simulink model "model_sample17a"  (R2017a)
settings: Solver=ode4  StartTime=0.0  StopTime=1000  FixedStep=1/30  RelTol=1e-3  EnableMultiTasking=on
settings Model: SimulationMode=external  ExtModeTrigDuration=200000  Creator=krecmich  LastModifiedBy=gurtnmar
settings DataIOCC: LimitDataPoints=on  SaveFormat=Array
settings OptimizationCC: ExpressionDepthLimit=2147483647  LifeSpan=1
settings DebuggingCC: UnderspecifiedInitializationDetection=Classic  MergeDetectMultiDrivingBlocksExec=none  SolverPrmCheckMsg=warning  StateNameClashWarn=warning  SFUnexpectedBacktrackingDiag=warning  SFNoUnconditionalDefaultTransitionDiag=warning  SFExecutionAtInitializationDiag=none
settings HardwareCC: ProdBitPerLong=64  ProdLargestAtomicFloat=None  ProdHWDeviceType=Intel->x86-64
settings ModelReferenceCC: PropagateSignalLabelsOutOfModel=off
settings SFSimCC: MATLABDynamicMemAlloc=off
settings RTWCC: SystemTargetFile=ert_linux.tlc  MakeCommand="make_rtw OPT_OPTS=\"-O2 -ggdb -Wall\" CC=aarch64-linux-gnu-gcc CPP=aarch64-linux-gnu-gcc"  TemplateMakefile=ert_linux.tmf  Description=Linux Embedded Coder
settings CodeAppCC: IgnoreCustomStorageClasses=off  CustomSymbolStrType=$N$R$M  InternalIdentifier=Classic
settings STFCustomTargetCC: TargetLangStandard=C99 (ISO)  ModelReferenceCompliant=off  CombineOutputUpdateFcns=on  ERTCustomFileBanners=on  RemoveResetFunc=on  MATLABClassNameForMDSCustomization=Simulink.SoftwareTarget.ERTCustomization  GRTInterface=off  SystemTargetFile=ert_linux.tlc
settings ERTTargetCC: TargetLangStandard=C99 (ISO)  MultiwordLength=2048  ModelReferenceCompliant=off  ParMdlRefBuildCompliant=off  CompOptLevelCompliant=off  ConcurrentExecutionCompliant=off  ERTFirstTimeCompliant=off  SupportContinuousTime=on  SupportNonInlinedSFcns=on  ModelStepFunctionPrototypeControlCompliant=off  CPPClassGenCompliant=off  UseToolchainInfoCompliant=off  ExtMode=on  ExtModeMexArgs='147.32.86.138'  ERTCustomFileTemplate=ert_linux_file_process.tlc  ConvertIfToSwitch=off  SuppressUnreachableDefaultCases=off
settings ConfigComp: CovMetricSettings=dw  CovHtmlReporting=on  CovSaveCumulativeToWorkspaceVar=on  CovSaveSingleToWorkspaceVar=on  CovExternalEMLEnable=off

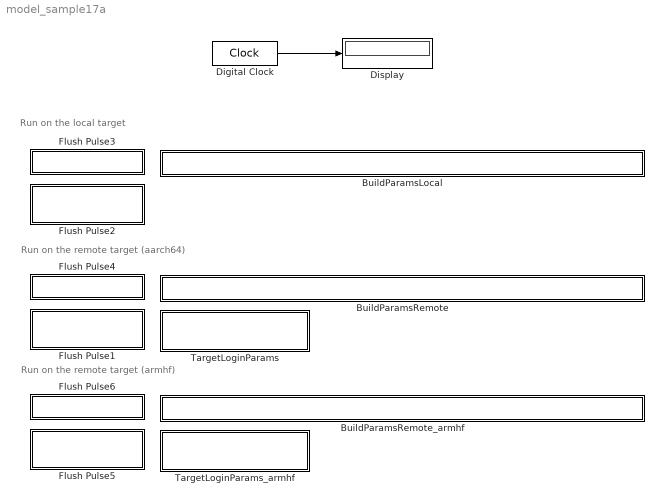
== system model_sample17a ==
  note: Run on the local target
  note: Run on the remote target (aarch64)
  note: Run on the remote target (armhf)
  BuildParamsLocal : Subsystem  mask{make_command='make_rtw OPT_OPTS="-O2 -ggdb -Wall" CC=gcc'}
      mask prompts: make_command "MakeCommand"
      mask Display: disp(get_param(gcb, 'make_command'));
  BuildParamsRemote : Subsystem  mask{make_command='make_rtw OPT_OPTS="-O2 -ggdb -Wall" CC=aarch64-linux-gnu-gcc CPP=aarch64-linux-gnu-gcc'}
      mask prompts: make_command "MakeCommand"
      mask Display: disp(get_param(gcb, 'make_command'));
  BuildParamsRemote_armhf : Subsystem  mask{make_command='make_rtw OPT_OPTS="-O2 -ggdb -Wall" CC=arm-linux-gnueabihf-gcc CPP=arm-linux-gnueabihf-gcc'}
      mask prompts: make_command "MakeCommand"
      mask Display: disp(get_param(gcb, 'make_command'));
  Digital Clock : DigitalClock
  Display : Display
  Flush Pulse1 : Subsystem
      settings: OpenFcn=|
      | % get the login credentials from the TargetLoginParams block
      | trgt_ip = get_param(strcat(gcs, '/TargetLoginParams'), 'trgt_ip_addr');
      | trgt_user = get_param(strcat(gcs, '/TargetLoginParams'), 'trgt_username');
      | 
      | % Set the IP address of the target
      | set_param(getActiveConfigSet(gcs), 'ExtModeMexArgs', trgt_ip);
      | 
      | system(['./run_model.sh ', get_param(bdroot(gcbh),'name'),' ',trgt_ip,' ',trgt_user]);
      mask Display: disp('Deploy and\nwait for connection')
  Flush Pulse2 : Subsystem
      settings: OpenFcn=|
      | configSet = getActiveConfigSet(gcs);
      | % Set the make command params
      | set_param( configSet, 'MakeCommand', '''make_rtw OPT_OPTS="-O2 -ggdb -Wall" CC=gcc''')
      | 
      | % Set the IP address of the target to the localhost
      | set_param(getActiveConfigSet(gcs), 'ExtModeMexArgs', '''127.0.0.1''')
      | 
      | system(['./run_model.sh ', get_param(bdroot(gcbh),'name')]);
      mask Display: disp('Deploy and\nwait for connection')
  Flush Pulse3 : Subsystem
      settings: OpenFcn=|
      | configSet = getActiveConfigSet(gcs);
      | % Set the make command params
      | set_param( configSet, 'MakeCommand', eval(get_param(strcat(gcs, '/BuildParamsLocal'), 'make_command')))
      | 
      | % Build the model
      | rtwbuild(gcs);
      mask Display: disp('Build')
  Flush Pulse4 : Subsystem
      settings: OpenFcn=|
      | configSet = getActiveConfigSet(gcs);
      | % Set the make command params
      | set_param( configSet, 'MakeCommand', eval(get_param(strcat(gcs, '/BuildParamsRemote'), 'make_command')))
      | 
      | % Build the model
      | rtwbuild(gcs);
      mask Display: disp('Build')
  Flush Pulse5 : Subsystem
      settings: OpenFcn=|
      | % get the login credentials from the TargetLoginParams block
      | trgt_ip = get_param(strcat(gcs, '/TargetLoginParams_armhf'), 'trgt_ip_addr');
      | trgt_user = get_param(strcat(gcs, '/TargetLoginParams_armhf'), 'trgt_username');
      | 
      | % Set the IP address of the target
      | set_param(getActiveConfigSet(gcs), 'ExtModeMexArgs', trgt_ip);
      | 
      | system(['./run_model.sh ', get_param(bdroot(gcbh),'name'),' ',trgt_ip,' ',trgt_user]);
      mask Display: disp('Deploy and\nwait for connection')
  Flush Pulse6 : Subsystem
      settings: OpenFcn=|
      | configSet = getActiveConfigSet(gcs);
      | % Set the make command params
      | set_param( configSet, 'MakeCommand', eval(get_param(strcat(gcs, '/BuildParamsRemote_armhf'), 'make_command')))
      | 
      | % Build the model
      | rtwbuild(gcs);
      mask Display: disp('Build')
  TargetLoginParams : Subsystem  mask{trgt_ip_addr='192.168.1.10', trgt_username='user'}
      mask prompts: trgt_ip_addr "Target IP address"; trgt_username "Target username"
      mask Display:
      | ip_addr = get_param(gcb, 'trgt_ip_addr');
      | user = get_param(gcb, 'trgt_username');
      | 
      | fprintf('IP addr:\t %s\n User:\t %s ', ip_addr, user);
  TargetLoginParams_armhf : Subsystem  mask{trgt_ip_addr='192.168.1.10', trgt_username='user'}
      mask prompts: trgt_ip_addr "Target IP address"; trgt_username "Target username"
      mask Display:
      | ip_addr = get_param(gcb, 'trgt_ip_addr');
      | user = get_param(gcb, 'trgt_username');
      | 
      | fprintf('IP addr:\t %s\n User:\t %s ', ip_addr, user);
  wires:
  Digital Clock/1 -> Display/1

== system model_sample17a/BuildParamsLocal ==

== system model_sample17a/BuildParamsRemote ==

== system model_sample17a/BuildParamsRemote_armhf ==

== system model_sample17a/Flush Pulse1 ==

== system model_sample17a/Flush Pulse2 ==

== system model_sample17a/Flush Pulse3 ==

== system model_sample17a/Flush Pulse4 ==

== system model_sample17a/Flush Pulse5 ==

== system model_sample17a/Flush Pulse6 ==

== system model_sample17a/TargetLoginParams ==

== system model_sample17a/TargetLoginParams_armhf ==
